simulink subsystem "invertMatrix"  (R2024b)
settings: Solver=VariableStepAuto  StartTime=0.0  StopTime=10.0  RelTol=1e-3
settings Model: Creator=ricca  LastModifiedBy=ricca

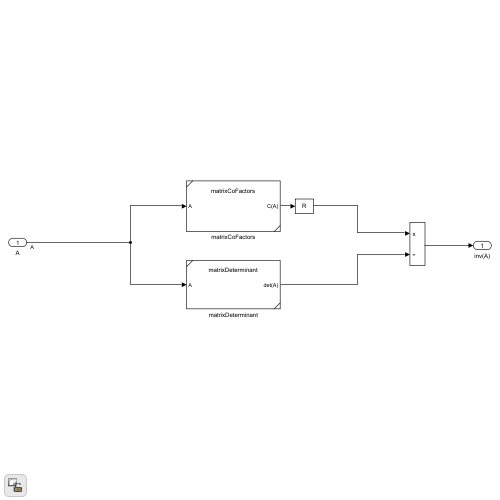
[thumbnail: Simulink's stored preview of the top-level diagram]
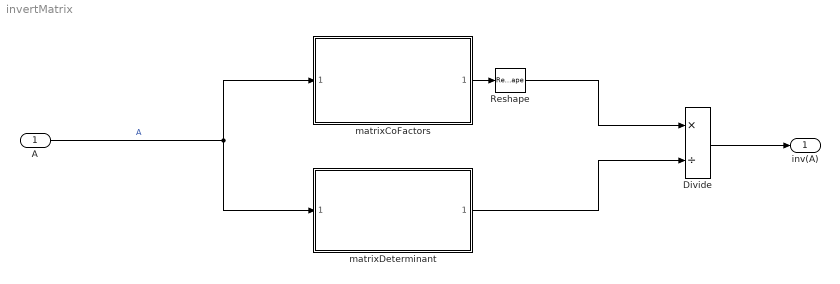
== system invertMatrix ==
  A : Inport
  Divide : Product  Inputs=*/
  Reshape : Reshape  OutputDimensionality=Customize  OutputDimensions=[3,3]
  matrixCoFactors : Subsystem  ReferencedSubsystem=matrixCoFactors
  matrixDeterminant : Subsystem  ReferencedSubsystem=matrixDeterminant
  inv(A) : Outport
  wires:
  A/1 -> matrixCoFactors/1, matrixDeterminant/1  "A"
  matrixCoFactors/1 -> Reshape/1
  matrixDeterminant/1 -> Divide/2
  Reshape/1 -> Divide/1
  Divide/1 -> inv(A)/1
